simulink model "BaseMotorSimulink"  (R2020a)
settings: Solver=VariableStepAuto  StartTime=0.0  StopTime=SimTime  FixedStep=solverTimeStep  RelTol=1e-3
InitFcn:
  | StartupScript
values from neighbouring files (symbols this model uses):
  CF = 1000.0    (= 1000)    [StartupScript.m]
  GearRatiob = 111.0    (= 111)    [StartupScript.m]
  Isat = 10.0    (= 10)    [StartupScript.m]
  Kb = 800.0    (= 800)    [StartupScript.m]
  Kdb = 1050    [StartupScript.m]
  Kib = 0    [StartupScript.m]
  Kmb = 23.4*1e-3    (= 0.0234)    [StartupScript.m]
  Kpb = 1000    [StartupScript.m]
  PidLim = 1024    [StartupScript.m]
  PidUCGain = 5/1024    (= 0.0048828125)    [StartupScript.m]
  r2d = 180/pi    (= 57.2957795131)    [StartupScript.m]
  sensorGain = 150.0    (= 150)    [StartupScript.m]
  Vsat = 18.0    (= 18)    [StartupScript.m]
libraries: cstblocks x4
settings Model: Creator=nisch  LastModifiedBy=nisch

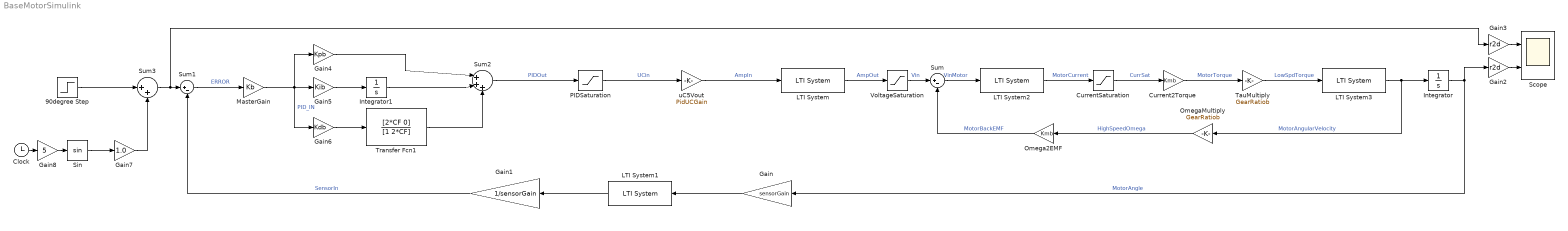
== system BaseMotorSimulink ==
  90degree Step : Step  Time=0  After=pi  SampleTime=0
  Clock : Clock
  Current2Torque : Gain  Gain=Kmb
  CurrentSaturation : Saturate  UpperLimit=Isat  LowerLimit=-Isat
  Gain : Gain  Gain=sensorGain
  Gain1 : Gain  Gain=1/sensorGain
  Gain2 : Gain  Gain=r2d
  Gain3 : Gain  Gain=r2d
  Gain4 : Gain  Gain=Kpb
  Gain5 : Gain  Gain=Kib
  Gain6 : Gain  Gain=Kdb
  Gain7 : Gain  Gain=1.0
  Gain8 : Gain  Gain=5
  Integrator : Integrator
  Integrator1 : Integrator
  LTI System : cstblocks/LTI System  sys=VoltageAmplifier  IC=[]
  LTI System1 : cstblocks/LTI System  sys=Hs  IC=[]
  LTI System2 : cstblocks/LTI System  sys=Electricalb  IC=[]
  LTI System3 : cstblocks/LTI System  sys=Mechanicalb  IC=[]
  MasterGain : Gain  Gain=Kb
  Omega2EMF : Gain  Gain=Kmb
  OmegaMultiply : Gain  Gain=GearRatiob
  PIDSaturation : Saturate  UpperLimit=PidLim  LowerLimit=-PidLim
  Scope : Scope  NumInputPorts=2
  Sin : Trigonometry
  Sum : Sum  Inputs=|+-
  Sum1 : Sum  Inputs=|+-
  Sum2 : Sum  Inputs=|+++
  Sum3 : Sum  Inputs=|++
  TauMultiply : Gain  Gain=GearRatiob
  Transfer Fcn1 : TransferFcn  Numerator=[2*CF 0]  Denominator=[1 2*CF]
  VoltageSaturation : Saturate  UpperLimit=Vsat  LowerLimit=-Vsat
  uC5Vout : Gain  Gain=PidUCGain
  wires:
  Sum/1 -> LTI System2/1  "VinMotor"
  Omega2EMF/1 -> Sum/2  "MotorBackEMF"
  LTI System3/1 -> Integrator/1, OmegaMultiply/1  "MotorAngularVelocity"
  Sum1/1 -> MasterGain/1  "ERROR"
  Integrator/1 -> Gain2/1, Gain/1  "MotorAngle"
  Gain/1 -> LTI System1/1
  LTI System1/1 -> Gain1/1
  Gain1/1 -> Sum1/2  "SensorIn"
  Gain2/1 -> Scope/2
  Gain3/1 -> Scope/1
  VoltageSaturation/1 -> Sum/1  "Vin"
  MasterGain/1 -> Gain6/1, Gain5/1, Gain4/1  "PID_IN"
  Gain5/1 -> Integrator1/1
  Gain6/1 -> Transfer Fcn1/1
  Sum2/1 -> PIDSaturation/1  "PIDOut"
  Gain4/1 -> Sum2/1
  Integrator1/1 -> Sum2/2
  Transfer Fcn1/1 -> Sum2/3
  LTI System2/1 -> CurrentSaturation/1  "MotorCurrent"
  CurrentSaturation/1 -> Current2Torque/1  "CurrSat"
  Current2Torque/1 -> TauMultiply/1  "MotorTorque"
  TauMultiply/1 -> LTI System3/1  "LowSpdTorque"
  OmegaMultiply/1 -> Omega2EMF/1  "HighSpeedOmega"
  Sum3/1 -> Gain3/1, Sum1/1
  90degree Step/1 -> Sum3/1
  Sin/1 -> Gain7/1
  Gain7/1 -> Sum3/2
  Clock/1 -> Gain8/1
  Gain8/1 -> Sin/1
  LTI System/1 -> VoltageSaturation/1  "AmpOut"
  PIDSaturation/1 -> uC5Vout/1  "UCin"
  uC5Vout/1 -> LTI System/1  "AmpIn"
